simulink model "BLDC_120deg_calibration_routine"  (R2024a)
settings: Solver=ode15s  StartTime=0.0  StopTime=2.25  RelTol=1e-3
model workspace (MAT data in the model file):
  t = 3
values from neighbouring files (symbols this model uses):
  D_m = 1e-3    (= 0.001)    [BLDC_Parameters.m]
  J_t = 1e-3    (= 0.001)    [BLDC_Parameters.m]
  L_ss = tau_s * r_s    (= 0.0003657)    [BLDC_Parameters.m]
  lambda_m = torque_const/(3*P/4)    (= 0.00985)    [BLDC_Parameters.m]
  P = 8    [BLDC_Parameters.m]
  r_s = r_pp/2    (= 0.345)    [BLDC_Parameters.m]
  R_vs = 1e6    (= 1000000)    [BLDC_Parameters.m]
  state1_tau = -1*mean(out.tau_state_1(end-5:end))*omega    [filter.m]
  state2_tau = -1*mean(out.tau_state_2(end-5:end))*omega    [filter.m]
  state3_tau = -1*mean(out.tau_state_3(end-5:end))*omega    [filter.m]
  state4_tau = -1*mean(out.tau_state_4(end-5:end))*omega    [filter.m]
  state5_tau = -1*mean(out.tau_state_5(end-5:end))*omega    [filter.m]
  state6_tau = -1*mean(out.tau_state_6(end-5:end))*omega    [filter.m]
  tau_s = 1.06e-3    (= 0.00106)    [BLDC_Parameters.m]
  V_bus = 12    [BLDC_Parameters.m]
undefined symbols (not defined in the file or in its folder): DiscIntNeverNeededParam, HallError1, HallError2, HallError3, WrappedHallError1
libraries: simulink x17, dspstat3 x6, spsMosfetLib x6, dspswit3 x5, spsSeriesRLCBranchLib x4, spsVoltageMeasurementLib x3, spsControlledCurrentSourceLib x3, slpidlib x1, spsPWMGeneratorDCDCLib x1, spsDCVoltageSourceLib x1, sps_lib x1
(part 1 of 2)
settings Model: Creator=matthewhasman  LastModifiedBy=matthewhasman

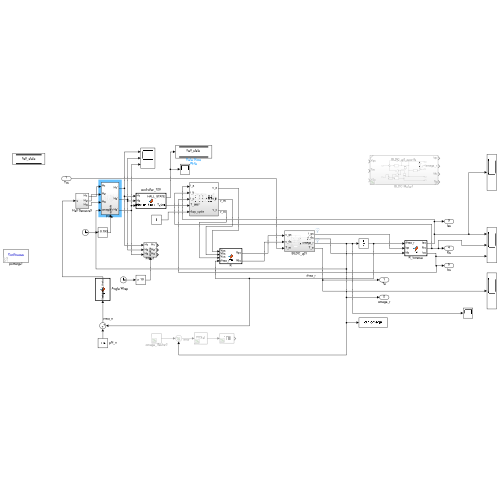
[thumbnail: Simulink's stored preview of the top-level diagram]
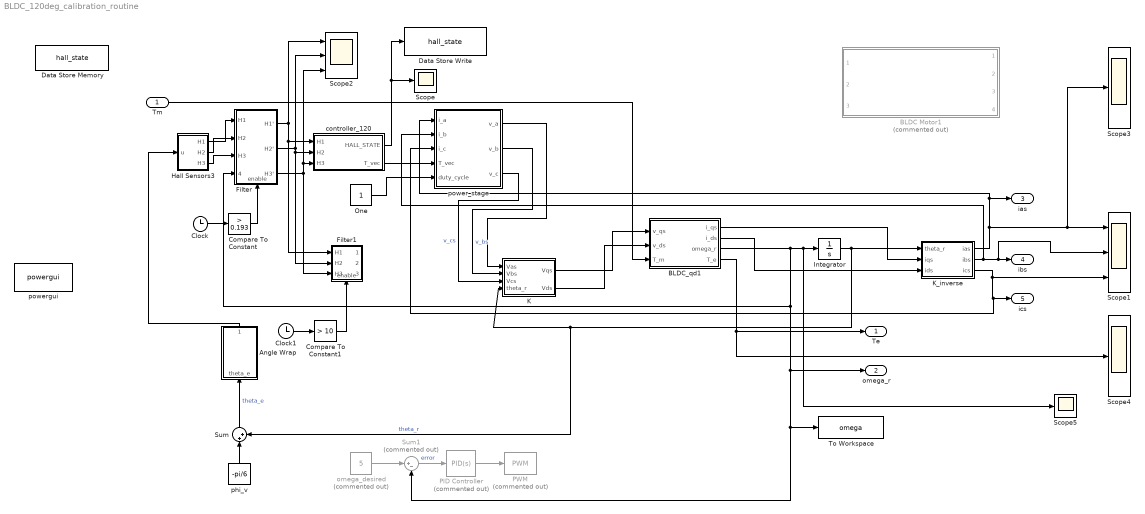
== system BLDC_120deg_calibration_routine ==
  Tm : Inport
  Angle Wrap : MATLAB Function  TreatAsAtomicUnit=on
  BLDC Motor1 : Subsystem  Commented=on  ReferencedSubsystem=BLDC_qd_coords
  BLDC_qd1 : Subsystem
  Clock : Clock
  Clock1 : Clock
  Compare To Constant : simulink/Logic and Bit Operations/Compare To Constant  relop=>  const=0.193  OutDataTypeStr=boolean
  Compare To Constant1 : simulink/Logic and Bit Operations/Compare To Constant  relop=>  const=10  OutDataTypeStr=boolean
  Data Store Memory : DataStoreMemory  DataStoreName=hall_state  WriteAfterWriteMsg=warning  InitialValue=-1  ShowAdditionalParam=off
  Data Store Write : DataStoreWrite  DataStoreName=hall_state  IndexOptions=Index vector (dialog)  Indices=1  OutputSizes=1
  Filter : Subsystem
      settings: PortSchema="{\"entries\":[{\"content\":{\"sides\":[{\"content\":{\"connectorIds\":[\"In1\",\"In2\",\"In3\",\"In4\"]},\"type\":\"ConnectorPlacement.EquallySpacedRectSide\",\"uuid\":\"41cc07ee-628c-4a70-9df5-9f0309ace514\"},{\"content\":{\"connectorIds\":[\"Out1\",\"Out2\",\"Out3\"],\"side\":\"RIGHT\"},\"type\":\"ConnectorPlacement.EquallySpacedRectSide\",\"uuid\":\"f15fe452-14eb-427f-ab3a-fd71ce3a6850\"},{\"content\":{\"side\":\"TOP\"},\"type\":\"ConnectorPlacement.EquallySpacedRectSide\",\"uuid\":\"a8bc91a7-4d9a-483b-b43c-6e71d37ef696\"},{\"content\":{\"connectorIds\":[\"In5\"],\"side\":\"BOTTOM\"},\"type\":\"ConnectorPlacement.EquallySpacedRectSide\",\"uuid\":\"b72df871-072d-40c5-aee7-b72e6fa3c48e\"}]},\"type\":\"ConnectorPlacement.EquallySpacedConnector\",\"uuid\":\"b89763df-ec25-48a8-941f-c6d30f9b0f80\"}],\"packageUris\":[\"http://schema.mathworks.com/mf0/Connector/R2020b\"],\"version\":\"1.0\"}"
  Filter1 : Subsystem
      settings: PortSchema="{\"entries\":[{\"content\":{\"sides\":[{\"content\":{\"connectorIds\":[\"In1\",\"In2\",\"In3\"]},\"type\":\"ConnectorPlacement.EquallySpacedRectSide\",\"uuid\":\"41cc07ee-628c-4a70-9df5-9f0309ace514\"},{\"content\":{\"connectorIds\":[\"Out1\",\"Out2\",\"Out3\"],\"side\":\"RIGHT\"},\"type\":\"ConnectorPlacement.EquallySpacedRectSide\",\"uuid\":\"f15fe452-14eb-427f-ab3a-fd71ce3a6850\"},{\"content\":{\"side\":\"TOP\"},\"type\":\"ConnectorPlacement.EquallySpacedRectSide\",\"uuid\":\"a8bc91a7-4d9a-483b-b43c-6e71d37ef696\"},{\"content\":{\"connectorIds\":[\"In4\"],\"side\":\"BOTTOM\"},\"type\":\"ConnectorPlacement.EquallySpacedRectSide\",\"uuid\":\"b72df871-072d-40c5-aee7-b72e6fa3c48e\"}]},\"type\":\"ConnectorPlacement.EquallySpacedConnector\",\"uuid\":\"b89763df-ec25-48a8-941f-c6d30f9b0f80\"}],\"packageUris\":[\"http://schema.mathworks.com/mf0/Connector/R2020b\"],\"version\":\"1.0\"}"
  Hall Sensors3 : Subsystem
  Integrator : Integrator
  K : MATLAB Function  TreatAsAtomicUnit=on
  K_inverse : MATLAB Function  TreatAsAtomicUnit=on
  One : Constant  OutDataTypeStr=Inherit: Inherit via back propagation
  PID Controller : slpidlib/PID Controller  Commented=on  Controller=PID  Form=Parallel  TimeDomain=Continuous-time  UseExternalTs=off  SampleTime=-1  IntegratorMethod=Forward Euler  FilterMethod=Forward Euler  ControllerParametersSource=internal  P=8  I=5  UseKiTs=off  D=1  UseExternalDerivativeSource=off  N=100  UseFilter=on  TunerSelectOption=Transfer Function Based (PID Tuner App)  InitialConditionSource=internal  InitialConditionForIntegrator=0  InitialConditionForFilter=0  DifferentiatorICPrevScaledInput=0  ExternalReset=none  TrackingMode=off  Kt=1  LimitOutput=off  SatLimitsSource=internal  UpperSaturationLimit=inf  LowerSaturationLimit=-inf  LinearizeAsGain=on  AntiWindupMode=none  Kb=1  LimitIntegrator=off  UpperIntegratorSaturationLimit=inf  LowerIntegratorSaturationLimit=-inf  POutMin=[]  POutMax=[]  IOutMin=[]  IOutMax=[]  DOutMin=[]  DOutMax=[]  NOutMin=[]  NOutMax=[]  SumOutMin=[]  SumOutMax=[]  SaturationOutMin=[]  SaturationOutMax=[]  PParamMin=[]  PParamMax=[]  IParamMin=[]  IParamMax=[]  DParamMin=[]  DParamMax=[]  NParamMin=[]  NParamMax=[]  KbParamMin=[]  KbParamMax=[]  KtParamMin=[]  KtParamMax=[]  KbOutMin=[]  KbOutMax=[]  KtOutMin=[]  KtOutMax=[]  IntegratorOutMin=[]  IntegratorOutMax=[]  FilterOutMin=[]  FilterOutMax=[]  SumI1OutMin=[]  SumI1OutMax=[]  SumI2OutMin=[]  SumI2OutMax=[]  SumI3OutMin=[]  SumI3OutMax=[]  SumI4OutMin=[]  SumI4OutMax=[]  SumDOutMin=[]  SumDOutMax=[]  DifferentiatorOutMin=[]  DifferentiatorOutMax=[]  FilterDiffOutCoefMin=[]  FilterDiffOutCoefMax=[]  ReciprocalOutMin=[]  ReciprocalOutMax=[]  SumDenOutMin=[]  SumDenOutMax=[]  SumNumOutMin=[]  SumNumOutMax=[]  DivideOutMin=[]  DivideOutMax=[]  UdiffTsProdOutMin=[]  UdiffTsProdOutMax=[]  NTsProdOutMin=[]  NTsProdOutMax=[]  UintegralTsProdOutMin=[]  UintegralTsProdOutMax=[]  UngainTsProdOutMin=[]  UngainTsProdOutMax=[]  ClampingZeroOutDataTypeStr=Inherit: Inherit via back propagation  ClampingZeroOutMin=[]  ClampingZeroOutMax=[]  FilterDenConstantOutDataTypeStr=Inherit: Inherit via back propagation  FilterDenConstantOutMin=[]  FilterDenConstantOutMax=[]  PCopyOutDataTypeStr=Inherit: Inherit via back propagation  PCopyOutMin=[]  PCopyOutMax=[]  NCopyOutDataTypeStr=Inherit: Inherit via back propagation  NCopyOutMin=[]  NCopyOutMax=[]  IntegratorContinuousStateAttributes=''  IntegratorStateMustResolveToSignalObject=off  IntegratorRTWStateStorageClass=Auto  FilterContinuousStateAttributes=''  FilterStateMustResolveToSignalObject=off  FilterRTWStateStorageClass=Auto  ParallelPVariant=InternalParameters  IdealPVariant=Disabled  IVariant=InternalParameters  DVariant=InternalParameters  IntegratorVariant=Continuous  SatVariant=Disabled  AWVariant=Passthrough  PCopyVariant=Disabled  TRVariant=Disabled  FdbkBlocksVariant=Forward  IdealPFdbkVariant=Disabled  SatFdbkVariant=Disabled  DerivativeFilterVariant=ContFilter  NVariant=InternalParameters  NCopyVariant=Disabled  FilterICVariant=InternalICsFilter  IntegratorICVariant=InternalICs  ExternalResetVariant=Disabled  TRSumVariant=Passthrough  SumFdbkVariant=Disabled  SumVariant=Sum_PID  TsampFilterVariant=InternalTs  TsampNgainVariant=Passthrough  TsampIntegralVariant=Disabled_SignalSpec  ExternalSaturationOutDataTypeStr=Inherit: Same as second input  DerivativeSourceVariant=ErrorSignal
  PWM : simulink/Discontinuities/PWM  Commented=on  DisableCoverage=on  Period=0.0001  InitialDelay=0  DisallowZeroDutyCycle=off  RunAtFixedTimeIntervals=off  SampleTime=0.1
  Scope{,3..5} (4 alike) : Scope
  Scope1 : Scope  NumInputPorts=3
  Scope2 : Scope  NumInputPorts=3
  Sum : Sum  Inputs=|++
  Sum1 : Sum  Commented=on  Inputs=|+-
  To Workspace : ToWorkspace  VariableName=omega  SampleTime=-1
  controller_120 : MATLAB Function  TreatAsAtomicUnit=on
  omega_desired : Constant  Commented=on  Value=5
  phi_v : Constant  Value=-pi/6
  power_stage : Subsystem
  powergui : sps_lib/powergui  Priority=1  SimulationMode=Continuous  SampleTime=50e-6  frequency=60  Iterations=50  frequencyindice=0  Pbase=100e6  ErrMax=1e-4  UnitsV=kV  UnitsW=MW  buscounter=0  FunctionMessages=off  echomessages=off  EnableUseOfTLC=off  CurrentSourceSwitches=off  DisableSnubberDevices=off  DisableRonSwitches=off  DisableVfSwitches=off  DisplayEquations=off  AutomaticDiscreteSolvers=off  SolverType=Tustin/Backward Euler (TBE)  Interpol=off  ExternalGateDelay=off  methode=off  Ts=100  x0status=blocks  SPID=on  SwTol=0  HookPort=off  NonlinearTolerance=1e-4  nMaxIteration=100  ContinueOnMaxIteration=off  RestoreLinks=warning  ResistiveCurrentMeasurement=off  Frange=[0:2:500]  Ylog=off  Xlog=on  ShowGrid=off  save=off  variable=ZData  structure=0  ZoomFFT=off  StartTime=0.0  cycles=1  DisplayStyle=1  fundamental=60  FreqAxis=off  MaxFrequency=1000  frequencyindicesteady=1  RmsSteady=1  display=off
  Te : Outport
  omega_r : Outport  Port=2
  ias : Outport  Port=3
  ibs : Outport  Port=4
  ics : Outport  Port=5
  wires:
  Integrator/1 -> K_inverse/1(theta_r), K/4(theta_r), Sum/2  "theta_r"
  BLDC_qd1/1(i_qs) -> K_inverse/2(iqs)
  BLDC_qd1/2(i_ds) -> K_inverse/3(ids)
  K/1(Vqs) -> BLDC_qd1/1(v_qs)
  Tm/1 -> BLDC_qd1/3(T_m)
  phi_v/1 -> Sum/1
  omega_desired/1 -> Sum1/1
  Sum1/1 -> PID Controller/1  "error"
  PID Controller/1 -> PWM/1
  K/2(Vds) -> BLDC_qd1/2(v_ds)
  Sum/1 -> Angle Wrap/1(theta_e)  "theta_e"
  BLDC_qd1/3(omega_r) -> Filter/4(omega_r), omega_r/1, To Workspace/1, Sum1/2, Scope5/1, Integrator/1
  BLDC_qd1/4(T_e) -> Scope4/1, Te/1
  K_inverse/1(ias) -> ias/1, power_stage/1(i_a), Scope3/1, Scope1/1
  K_inverse/2(ibs) -> power_stage/2(i_b), Scope1/2, ibs/1
  K_inverse/3(ics) -> power_stage/3(i_c), ics/1, Scope1/3
  controller_120/2(T_vec) -> power_stage/4(T_vec)
  power_stage/1(v_a) -> K/1(Vas)
  power_stage/2(v_b) -> K/2(Vbs)  "v_bs"
  power_stage/3(v_c) -> K/3(Vcs)  "v_cs"
  Angle Wrap/1(wrapped_theta) -> Hall Sensors3/1(u)
  Hall Sensors3/1(H1) -> Filter/1(H1)
  Hall Sensors3/2(H2) -> Filter/2(H2)
  Hall Sensors3/3(H3) -> Filter/3(H3)
  Compare To Constant/1 -> Filter/5(enable)
  Filter/1(H1') -> Scope2/1, Filter1/1(H1), controller_120/1(H1)
  Filter/2(H2') -> Scope2/2, Filter1/2(H2), controller_120/2(H2)
  Filter/3(H3') -> Scope2/3, controller_120/3(H3), Filter1/3(H3)
  Clock/1 -> Compare To Constant/1
  controller_120/1(HALL_STATE) -> Scope/1, Data Store Write/1
  One/1 -> power_stage/5(duty_cycle)
  Compare To Constant1/1 -> Filter1/4(enable)
  Clock1/1 -> Compare To Constant1/1

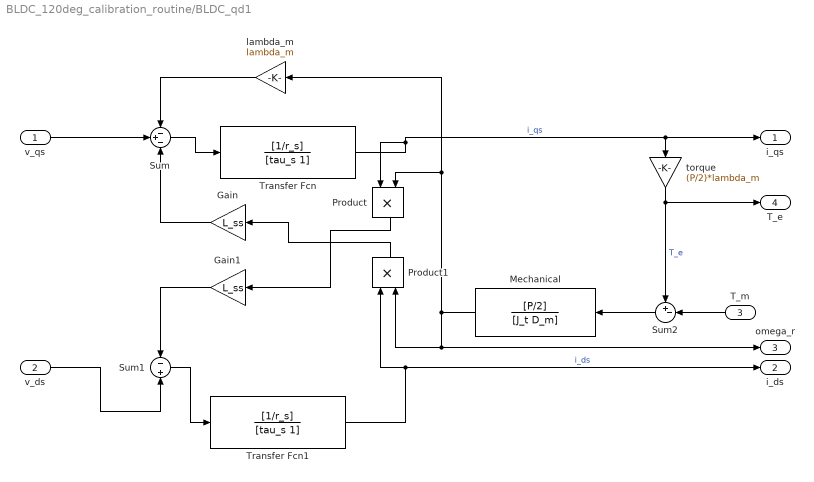
== system BLDC_120deg_calibration_routine/BLDC_qd1 ==
  v_qs : Inport
  v_ds : Inport  Port=2
  T_m : Inport  Port=3
  Gain : Gain  Gain=L_ss
  Gain1 : Gain  Gain=L_ss
  Mechanical : TransferFcn  Numerator=[P/2]  Denominator=[J_t D_m]
  Product : Product
  Product1 : Product
  Sum : Sum  Inputs=-+-
  Sum1 : Sum  Inputs=-+
  Sum2 : Sum  Inputs=+-|
  Transfer Fcn : TransferFcn  Numerator=[1/r_s]  Denominator=[tau_s 1]
  Transfer Fcn1 : TransferFcn  Numerator=[1/r_s]  Denominator=[tau_s 1]
  lambda_m : Gain  Gain=lambda_m
  torque : Gain  Gain=(P/2)*lambda_m
  i_qs : Outport
  i_ds : Outport  Port=2
  omega_r : Outport  Port=3
  T_e : Outport  Port=4
  wires:
  T_m/1 -> Sum2/2
  Sum1/1 -> Transfer Fcn1/1
  Gain1/1 -> Sum1/1
  Product1/1 -> Gain/1
  Transfer Fcn1/1 -> i_ds/1, Product1/1  "i_ds"
  Mechanical/1 -> lambda_m/1, Product/2, omega_r/1, Product1/2
  torque/1 -> T_e/1, Sum2/1  "T_e"
  v_ds/1 -> Sum1/2
  Transfer Fcn/1 -> i_qs/1, torque/1, Product/1  "i_qs"
  Product/1 -> Gain1/1
  Gain/1 -> Sum/3
  v_qs/1 -> Sum/2
  Sum/1 -> Transfer Fcn/1
  Sum2/1 -> Mechanical/1
  lambda_m/1 -> Sum/1

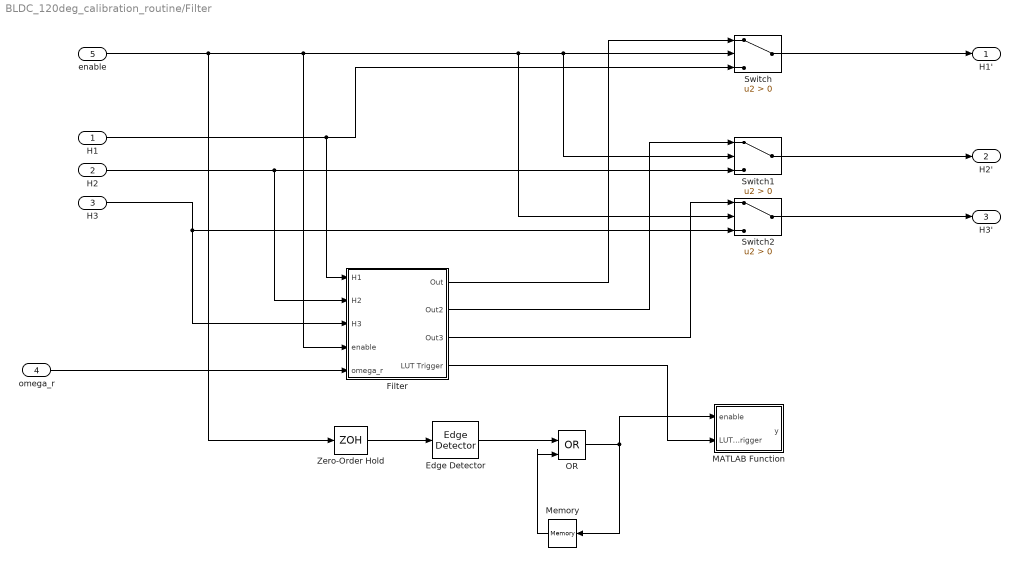
== system BLDC_120deg_calibration_routine/Filter ==
  H1 : Inport
  H2 : Inport  Port=2
  H3 : Inport  Port=3
  omega_r : Inport  Port=4
  enable : Inport  Port=5
  Edge Detector : dspswit3/Edge Detector  InputProcessing=Columns as channels (frame based)
  Filter : Subsystem
  MATLAB Function : MATLAB Function  TreatAsAtomicUnit=on
  Memory : Memory
  OR : Logic  Operator=OR  IconShape=distinctive  AllPortsSameDT=off  OutDataTypeStr=boolean
  Switch : Switch  Criteria=u2 > Threshold  SaturateOnIntegerOverflow=off  InputSameDT=off
  Switch1 : Switch  Criteria=u2 > Threshold  SaturateOnIntegerOverflow=off  InputSameDT=off
  Switch2 : Switch  Criteria=u2 > Threshold  SaturateOnIntegerOverflow=off  InputSameDT=off
  Zero-Order Hold : ZeroOrderHold  SampleTime=-1
  H1' : Outport
  H2' : Outport  Port=2
  H3' : Outport  Port=3
  wires:
  H1/1 -> Switch/3, Filter/1(H1)
  H2/1 -> Filter/2(H2), Switch1/3
  H3/1 -> Switch2/3, Filter/3(H3)
  enable/1 -> Switch2/2, Switch1/2, Switch/2, Filter/4(enable), Zero-Order Hold/1
  Switch/1 -> H1'/1
  Switch1/1 -> H2'/1
  Switch2/1 -> H3'/1
  Filter/1(Out) -> Switch/1
  Filter/2(Out2) -> Switch1/1
  Filter/3(Out3) -> Switch2/1
  omega_r/1 -> Filter/5(omega_r)
  Edge Detector/1 -> OR/1
  Zero-Order Hold/1 -> Edge Detector/1
  OR/1 -> MATLAB Function/1(enable), Memory/1
  Memory/1 -> OR/2
  Filter/4(LUT Trigger) -> MATLAB Function/2(LUT_Trigger)

== system BLDC_120deg_calibration_routine/Filter1 ==
  H1 : Inport
  H2 : Inport  Port=2
  H3 : Inport  Port=3
  enable : Inport  Port=4
  Filter : Subsystem
  Switch : Switch  Criteria=u2 > Threshold  SaturateOnIntegerOverflow=off  InputSameDT=off
  Switch1 : Switch  Criteria=u2 > Threshold  SaturateOnIntegerOverflow=off  InputSameDT=off
  Switch2 : Switch  Criteria=u2 > Threshold  SaturateOnIntegerOverflow=off  InputSameDT=off
  H1' : Outport
  H2' : Outport  Port=2
  H3' : Outport  Port=3
  wires:
  H1/1 -> Switch/3, Filter/1(H1)
  H2/1 -> Filter/2(H2), Switch1/3
  H3/1 -> Switch2/3, Filter/3(H3)
  enable/1 -> Filter/4(enable), Switch2/2, Switch1/2, Switch/2
  Switch/1 -> H1'/1
  Switch1/1 -> H2'/1
  Switch2/1 -> H3'/1
  Filter/1(Out) -> Switch/1
  Filter/2(Out2) -> Switch1/1
  Filter/3(Out3) -> Switch2/1

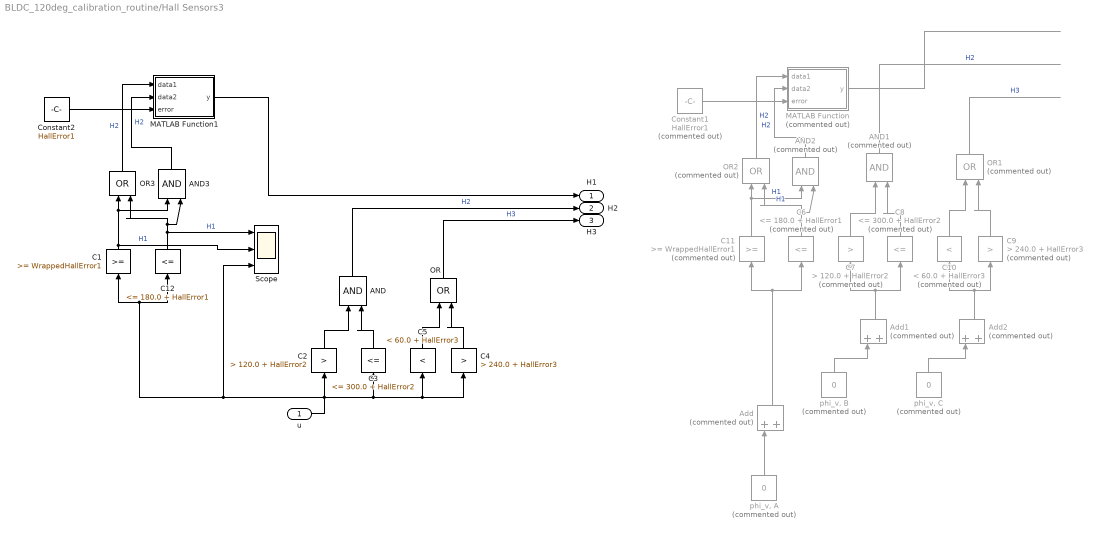
== system BLDC_120deg_calibration_routine/Hall Sensors3 ==
  u : Inport
  AND : Logic  IconShape=distinctive  AllPortsSameDT=off  OutDataTypeStr=boolean
  AND1 : Logic  Commented=on  IconShape=distinctive  AllPortsSameDT=off  OutDataTypeStr=boolean
  AND2 : Logic  Commented=on  IconShape=distinctive  AllPortsSameDT=off  OutDataTypeStr=boolean
  AND3 : Logic  IconShape=distinctive  AllPortsSameDT=off  OutDataTypeStr=boolean
  Add : Sum  Commented=on
  Add1 : Sum  Commented=on
  Add2 : Sum  Commented=on
  C1 : simulink/Logic and Bit Operations/Compare To Constant  relop=>=  const=WrappedHallError1  OutDataTypeStr=boolean
  C10 : simulink/Logic and Bit Operations/Compare To Constant  Commented=on  relop=<  const=60.0 + HallError3  OutDataTypeStr=boolean
  C11 : simulink/Logic and Bit Operations/Compare To Constant  Commented=on  relop=>=  const=WrappedHallError1  OutDataTypeStr=boolean
  C12 : simulink/Logic and Bit Operations/Compare To Constant  relop=<=  const=180.0 + HallError1  OutDataTypeStr=boolean
  C2 : simulink/Logic and Bit Operations/Compare To Constant  relop=>  const=120.0 + HallError2  OutDataTypeStr=boolean
  C3 : simulink/Logic and Bit Operations/Compare To Constant  relop=<=  const=300.0 + HallError2  OutDataTypeStr=boolean
  C4 : simulink/Logic and Bit Operations/Compare To Constant  relop=>  const=240.0 + HallError3  OutDataTypeStr=boolean
  C5 : simulink/Logic and Bit Operations/Compare To Constant  relop=<  const=60.0 + HallError3  OutDataTypeStr=boolean
  C6 : simulink/Logic and Bit Operations/Compare To Constant  Commented=on  relop=<=  const=180.0 + HallError1  OutDataTypeStr=boolean
  C7 : simulink/Logic and Bit Operations/Compare To Constant  Commented=on  relop=>  const=120.0 + HallError2  OutDataTypeStr=boolean
  C8 : simulink/Logic and Bit Operations/Compare To Constant  Commented=on  relop=<=  const=300.0 + HallError2  OutDataTypeStr=boolean
  C9 : simulink/Logic and Bit Operations/Compare To Constant  Commented=on  relop=>  const=240.0 + HallError3  OutDataTypeStr=boolean
  Constant1 : Constant  Commented=on  Value=HallError1
  Constant2 : Constant  Value=HallError1
  MATLAB Function : MATLAB Function  Commented=on  TreatAsAtomicUnit=on
  MATLAB Function1 : MATLAB Function  TreatAsAtomicUnit=on
  OR : Logic  Operator=OR  IconShape=distinctive  AllPortsSameDT=off  OutDataTypeStr=boolean
  OR1 : Logic  Commented=on  Operator=OR  IconShape=distinctive  AllPortsSameDT=off  OutDataTypeStr=boolean
  OR2 : Logic  Commented=on  Operator=OR  IconShape=distinctive  AllPortsSameDT=off  OutDataTypeStr=boolean
  OR3 : Logic  Operator=OR  IconShape=distinctive  AllPortsSameDT=off  OutDataTypeStr=boolean
  Scope : Scope  NumInputPorts=3
  "phi_v, A" : Constant  Commented=on  Value=0
  "phi_v, B" : Constant  Commented=on  Value=0
  "phi_v, C" : Constant  Commented=on  Value=0
  H1 : Outport
  H2 : Outport  Port=2
  H3 : Outport  Port=3
  wires:
  C5/1 -> OR/1
  AND/1 -> H2/1  "H2"
  C4/1 -> OR/2
  C3/1 -> AND/2
  C2/1 -> AND/1
  OR/1 -> H3/1  "H3"
  Add1/1 -> C8/1, C7/1
  "phi_v, C"/1 -> Add2/1
  "phi_v, B"/1 -> Add1/1
  C10/1 -> OR1/1
  ? -> Add2/2, Add1/2, Add/2
  OR2/1 -> MATLAB Function/1(data1)  "H2"
  "phi_v, A"/1 -> Add/1
  C9/1 -> OR1/2
  Add/1 -> C6/1, C11/1
  C7/1 -> AND1/1
  Add2/1 -> C10/1, C9/1
  Constant1/1 -> MATLAB Function/3(error)
  OR1/1 -> ?  "H3"
  AND1/1 -> ?  "H2"
  C6/1 -> AND2/2, OR2/2  "H1"
  AND2/1 -> MATLAB Function/2(data2)  "H2"
  MATLAB Function/1(y) -> ?
  C11/1 -> AND2/1, OR2/1  "H1"
  C8/1 -> AND1/2
  u/1 -> Scope/3, C12/1, C1/1, C2/1, C5/1, C4/1, C3/1
  OR3/1 -> MATLAB Function1/1(data1)  "H2"
  Constant2/1 -> MATLAB Function1/3(error)
  C1/1 -> AND3/1, OR3/1, Scope/2  "H1"
  C12/1 -> AND3/2, OR3/2, Scope/1  "H1"
  AND3/1 -> MATLAB Function1/2(data2)  "H2"
  MATLAB Function1/1(y) -> H1/1

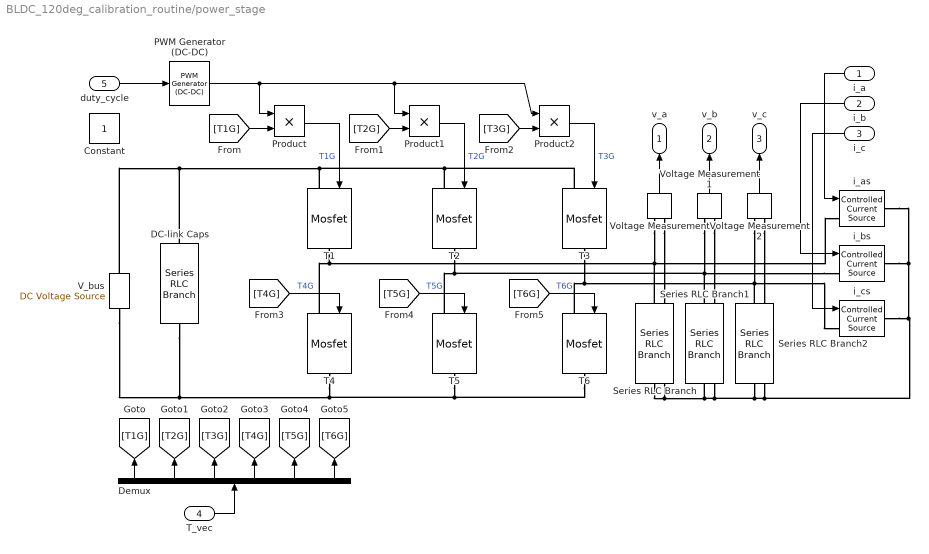
== system BLDC_120deg_calibration_routine/power_stage ==
  i_a : Inport
  i_b : Inport  Port=2
  i_c : Inport  Port=3
  T_vec : Inport  Port=4
  duty_cycle : Inport  Port=5
  Constant : Constant
  DC-link Caps : spsSeriesRLCBranchLib/Series RLC Branch  LConnTagsString=__new0  RConnTagsString=__new0  BranchType=RC  Resistance=1e-6  Inductance=0  SetiL0=off  InitialCurrent=0  Capacitance=100e-6  Setx0=off  InitialVoltage=0  Measurements=None
  Demux : Demux  Outputs=6
  PWM Generator (DC-DC) : spsPWMGeneratorDCDCLib/PWM Generator (DC-DC)  Fsw=f_SW_Hz  Ts=0
  Product : Product
  Product1 : Product
  Product2 : Product
  Series RLC Branch : spsSeriesRLCBranchLib/Series RLC Branch  LConnTagsString=__new0  RConnTagsString=__new0  BranchType=R  Resistance=R_vs  Inductance=0  SetiL0=off  InitialCurrent=0  Capacitance=inf  Setx0=off  InitialVoltage=0  Measurements=None
  Series RLC Branch1 : spsSeriesRLCBranchLib/Series RLC Branch  LConnTagsString=__new0  RConnTagsString=__new0  BranchType=R  Resistance=R_vs  Inductance=0  SetiL0=off  InitialCurrent=0  Capacitance=inf  Setx0=off  InitialVoltage=0  Measurements=None
  Series RLC Branch2 : spsSeriesRLCBranchLib/Series RLC Branch  LConnTagsString=__new0  RConnTagsString=__new0  BranchType=R  Resistance=R_vs  Inductance=0  SetiL0=off  InitialCurrent=0  Capacitance=inf  Setx0=off  InitialVoltage=0  Measurements=None
  T{1..6} (6 alike) : spsMosfetLib/Mosfet  Ron=R_dsON_Ohm  Lon=0  Rd=0.01  Vfd=0.7  IC=0  Rs=1e5  Cs=inf  Measurements=off
  V_bus : spsDCVoltageSourceLib/DC Voltage Source  Amplitude=V_bus  Measurements=None
  Voltage Measurement : spsVoltageMeasurementLib/Voltage Measurement  PhasorSimulation=off  OutputType=Complex  PSBequivalent=0
  Voltage Measurement1 : spsVoltageMeasurementLib/Voltage Measurement  PhasorSimulation=off  OutputType=Complex  PSBequivalent=0
  Voltage Measurement2 : spsVoltageMeasurementLib/Voltage Measurement  PhasorSimulation=off  OutputType=Complex  PSBequivalent=0
  i_as : spsControlledCurrentSourceLib/Controlled Current Source  Initialize=on  Source_Type=AC  Amplitude=0  Phase=0  Frequency=0  Measurements=None
  i_bs : spsControlledCurrentSourceLib/Controlled Current Source  Initialize=on  Source_Type=AC  Amplitude=0  Phase=0  Frequency=0  Measurements=None
  i_cs : spsControlledCurrentSourceLib/Controlled Current Source  Initialize=on  Source_Type=AC  Amplitude=0  Phase=0  Frequency=0  Measurements=None
  v_a : Outport
  v_b : Outport  Port=2
  v_c : Outport  Port=3
  wires:
  T_vec/1 -> Demux/1
  Product1/1 -> T2/1  "T2G"
  PWM Generator (DC-DC)/1 -> Product/1, Product2/1, Product1/1
  Demux/6 -> [T6G]
  [T4G] -> T4/1  "T4G"
  [T5G] -> T5/1  "T5G"
  Demux/4 -> [T4G]
  Voltage Measurement/1 -> v_a/1
  [T2G] -> Product1/2
  Voltage Measurement1/1 -> v_b/1
  Voltage Measurement2/1 -> v_c/1
  i_a/1 -> i_as/1
  Demux/1 -> [T1G]
  Demux/5 -> [T5G]
  [T6G] -> T6/1  "T6G"
  i_c/1 -> i_cs/1
  Product/1 -> T1/1  "T1G"
  [T3G] -> Product2/2
  i_b/1 -> i_bs/1
  Product2/1 -> T3/1  "T3G"
  Demux/2 -> [T2G]
  Demux/3 -> [T3G]
  [T1G] -> Product/2
  duty_cycle/1 -> PWM Generator (DC-DC)/1
  connections:
  i_bs/LConn1 -- Voltage Measurement1/LConn1 -- Series RLC Branch1/LConn1 -- T2/RConn1 -- T5/LConn1
  DC-link Caps/RConn1 -- V_bus/LConn1 -- T4/RConn1 -- T6/RConn1 -- T5/RConn1
  DC-link Caps/LConn1 -- V_bus/RConn1 -- T1/LConn1 -- T3/LConn1 -- T2/LConn1
  T4/LConn1 -- T1/RConn1 -- Voltage Measurement/LConn1 -- Series RLC Branch/LConn1 -- i_as/LConn1
  T3/RConn1 -- T6/LConn1 -- Voltage Measurement2/LConn1 -- Series RLC Branch2/LConn1 -- i_cs/LConn1
  Series RLC Branch/RConn1 -- Voltage Measurement/LConn2 -- i_bs/RConn1 -- i_as/RConn1 -- i_cs/RConn1 -- Voltage Measurement2/LConn2 -- Series RLC Branch2/RConn1 -- Voltage Measurement1/LConn2 -- Series RLC Branch1/RConn1

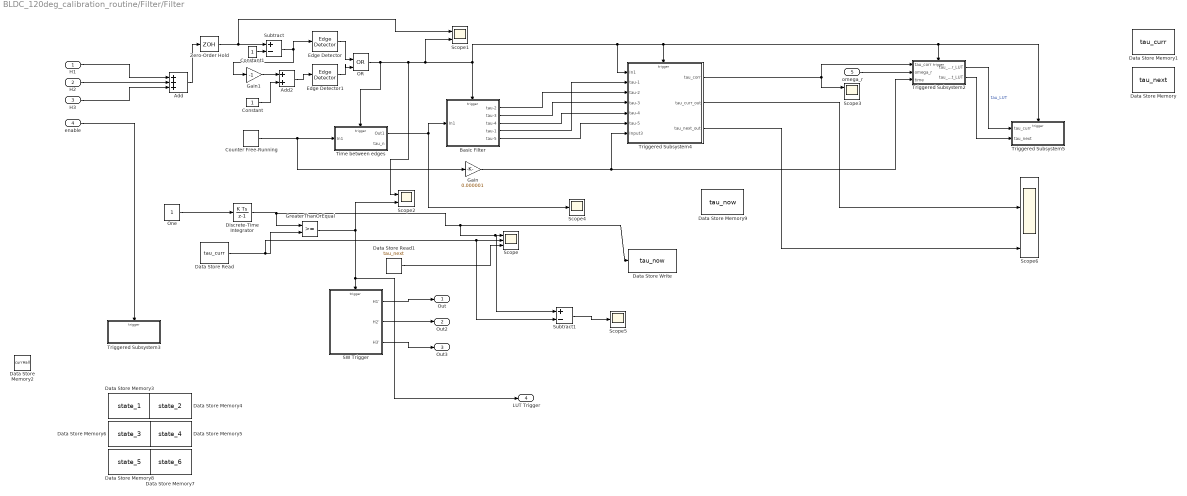
== system BLDC_120deg_calibration_routine/Filter/Filter ==
  H1 : Inport
  H2 : Inport  Port=2
  H3 : Inport  Port=3
  enable : Inport  Port=4
  omega_r : Inport  Port=5
  Add : Sum  Inputs=+++
  Add2 : Sum
  Basic Filter : Subsystem  TreatAsAtomicUnit=on
  Constant : Constant
  Constant1 : Constant
  Counter Free-Running : simulink/Sources/Counter Free-Running  NumBits=32  tsamp=0.000001
  Data Store Memory : DataStoreMemory  DataStoreName=tau_next  WriteAfterWriteMsg=warning  InitialValue=-1  ShowAdditionalParam=off
  Data Store Memory1 : DataStoreMemory  DataStoreName=tau_curr  WriteAfterWriteMsg=warning  InitialValue=0.001  ShowAdditionalParam=off
  Data Store Memory2 : DataStoreMemory  DataStoreName=currHall  WriteAfterWriteMsg=warning  InitialValue=1  ShowAdditionalParam=off
  Data Store Memory3 : DataStoreMemory  DataStoreName=state_1  WriteAfterWriteMsg=warning  ShowAdditionalParam=off
  Data Store Memory4 : DataStoreMemory  DataStoreName=state_2  WriteAfterWriteMsg=warning  ShowAdditionalParam=off
  Data Store Memory5 : DataStoreMemory  DataStoreName=state_4  WriteAfterWriteMsg=warning  ShowAdditionalParam=off
  Data Store Memory6 : DataStoreMemory  DataStoreName=state_3  WriteAfterWriteMsg=warning  ShowAdditionalParam=off
  Data Store Memory7 : DataStoreMemory  DataStoreName=state_6  WriteAfterWriteMsg=warning  ShowAdditionalParam=off
  Data Store Memory8 : DataStoreMemory  DataStoreName=state_5  WriteAfterWriteMsg=warning  ShowAdditionalParam=off
  Data Store Memory9 : DataStoreMemory  DataStoreName=tau_now  WriteAfterWriteMsg=warning  ShowAdditionalParam=off
  Data Store Read : DataStoreRead  DataStoreName=tau_curr  IndexOptions=Index vector (dialog)  Indices=1  OutputSizes=1
  Data Store Read1 : DataStoreRead  DataStoreName=tau_next  IndexOptions=Index vector (dialog)  Indices=1  OutputSizes=1
  Data Store Write : DataStoreWrite  DataStoreName=tau_now  IndexOptions=Index vector (dialog)  Indices=1  OutputSizes=1
  Discrete-Time Integrator : DiscreteIntegrator  SampleTime=1/1e6  ICPrevOutput=DiscIntNeverNeededParam  ICPrevScaledInput=DiscIntNeverNeededParam
  Edge Detector : dspswit3/Edge Detector  InputProcessing=Columns as channels (frame based)
  Edge Detector1 : dspswit3/Edge Detector  InputProcessing=Columns as channels (frame based)
  Gain : Gain  Gain=0.000001
  Gain1 : Gain  Gain=-1
  GreaterThanOrEqual : RelationalOperator  OutDataTypeStr=boolean  RndMeth=Simplest  InputSameDT=off
  OR : Logic  Operator=OR  IconShape=distinctive  AllPortsSameDT=off  OutDataTypeStr=boolean
  One : Constant  OutDataTypeStr=Inherit: Inherit via back propagation
  SW Trigger : Subsystem  Priority=2  TreatAsAtomicUnit=on
  Scope : Scope  NumInputPorts=3
  Scope1 : Scope  NumInputPorts=2
  Scope2 : Scope  NumInputPorts=2
  Scope3 : Scope  NumInputPorts=2
  Scope4 : Scope
  Scope5 : Scope
  Scope6 : Scope  NumInputPorts=4
  Subtract : Sum  Inputs=+-
  Subtract1 : Sum  Inputs=+-
  Time between edges : Subsystem  TreatAsAtomicUnit=on
  Triggered Subsystem2 : Subsystem  TreatAsAtomicUnit=on
  Triggered Subsystem3 : Subsystem  Priority=1  TreatAsAtomicUnit=on
  Triggered Subsystem4 : Subsystem  TreatAsAtomicUnit=on
  Triggered Subsystem5 : Subsystem  TreatAsAtomicUnit=on
  Zero-Order Hold : ZeroOrderHold  SampleTime=0.000001
  Out : Outport
  Out2 : Outport  Port=2
  Out3 : Outport  Port=3
  LUT Trigger : Outport  Port=4
  wires:
  Counter Free-Running/1 -> Gain/1, Time between edges/1(In1)
  Add/1 -> Zero-Order Hold/1
  Time between edges/1(Out1) -> Scope4/1, Basic Filter/1(In1)
  Edge Detector/1 -> OR/1
  Zero-Order Hold/1 -> Scope1/1, Subtract/1
  Subtract/1 -> Edge Detector/1, Gain1/1
  Constant1/1 -> Subtract/2
  Edge Detector1/1 -> OR/2
  Gain1/1 -> Add2/1
  Add2/1 -> Edge Detector1/1
  Constant/1 -> Add2/2
  H1/1 -> Add/1
  H2/1 -> Add/2
  H3/1 -> Add/3
  OR/1 -> Scope2/1, Scope1/2, Triggered Subsystem4/1(In1), Triggered Subsystem2/Trigger, Triggered Subsystem5/Trigger, Triggered Subsystem4/Trigger, Basic Filter/Trigger, Time between edges/Trigger
  Data Store Read/1 -> Subtract1/2, Scope/2, GreaterThanOrEqual/2
  GreaterThanOrEqual/1 -> LUT Trigger/1, SW Trigger/Trigger, Scope2/2
  SW Trigger/3(H3') -> Out3/1
  SW Trigger/2(H2') -> Out2/1
  SW Trigger/1(H1') -> Out/1
  Data Store Read1/1 -> Scope/3
  enable/1 -> Triggered Subsystem3/Trigger
  One/1 -> Discrete-Time Integrator/1
  Discrete-Time Integrator/1 -> Subtract1/1, Scope/1, Data Store Write/1, GreaterThanOrEqual/1
  Triggered Subsystem4/1(tau_corr) -> Triggered Subsystem2/1(tau_corr), Scope3/1
  Basic Filter/1(tau-2) -> Triggered Subsystem4/3(tau-2)
  Basic Filter/2(tau-3) -> Triggered Subsystem4/4(tau-3)
  Basic Filter/3(tau-4) -> Triggered Subsystem4/5(tau-4)
  Gain/1 -> Triggered Subsystem2/3(time), Triggered Subsystem4/7(Input3)
  Basic Filter/4(tau-1) -> Triggered Subsystem4/2(tau-1)
  Basic Filter/5(tau-5) -> Triggered Subsystem4/6(tau-5)
  Subtract1/1 -> Scope5/1
  omega_r/1 -> Triggered Subsystem2/2(omega_r)
  Triggered Subsystem4/2(tau_curr_out) -> Scope6/2
  Triggered Subsystem4/3(tau_next_out) -> Scope6/4
  Triggered Subsystem2/1(tau_curr_LUT) -> Triggered Subsystem5/1(tau_curr)  "tau_LUT"
  Triggered Subsystem2/2(tau_next_LUT) -> Triggered Subsystem5/2(tau_next)

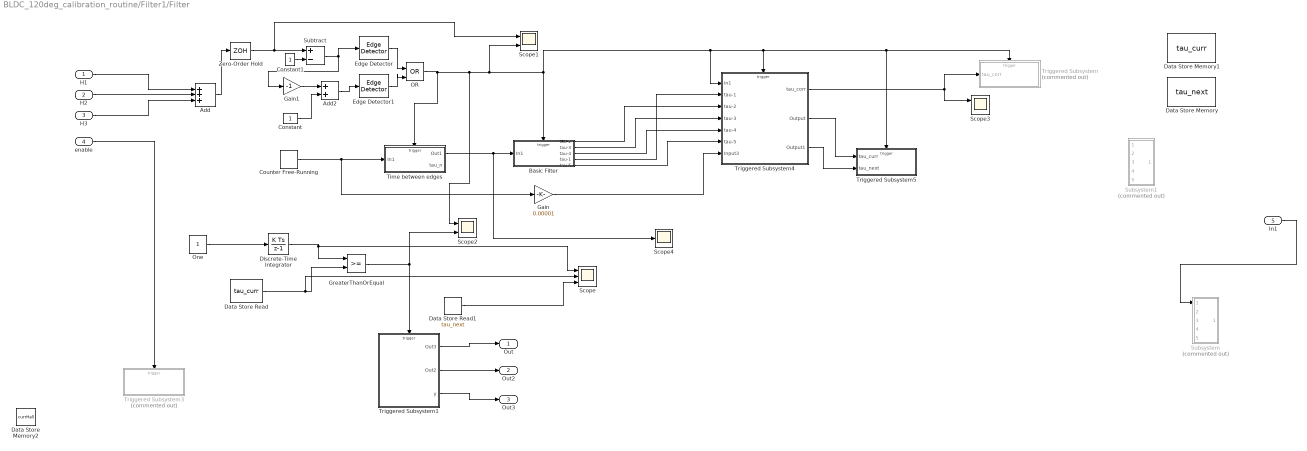
== system BLDC_120deg_calibration_routine/Filter1/Filter ==
  H1 : Inport
  H2 : Inport  Port=2
  H3 : Inport  Port=3
  enable : Inport  Port=4
  In1 : Inport  Port=5
  Add : Sum  Inputs=+++
  Add2 : Sum
  Basic Filter : Subsystem  TreatAsAtomicUnit=on
  Constant : Constant
  Constant1 : Constant
  Counter Free-Running : simulink/Sources/Counter Free-Running  NumBits=32  tsamp=0.000001
  Data Store Memory : DataStoreMemory  DataStoreName=tau_next  WriteAfterWriteMsg=warning  InitialValue=-1  ShowAdditionalParam=off
  Data Store Memory1 : DataStoreMemory  DataStoreName=tau_curr  WriteAfterWriteMsg=warning  InitialValue=0.001  ShowAdditionalParam=off
  Data Store Memory2 : DataStoreMemory  DataStoreName=currHall  WriteAfterWriteMsg=warning  InitialValue=1  ShowAdditionalParam=off
  Data Store Read : DataStoreRead  DataStoreName=tau_curr  IndexOptions=Index vector (dialog)  Indices=1  OutputSizes=1
  Data Store Read1 : DataStoreRead  DataStoreName=tau_next  IndexOptions=Index vector (dialog)  Indices=1  OutputSizes=1
  Discrete-Time Integrator : DiscreteIntegrator  SampleTime=1/1e5  ICPrevOutput=DiscIntNeverNeededParam  ICPrevScaledInput=DiscIntNeverNeededParam
  Edge Detector : dspswit3/Edge Detector  InputProcessing=Columns as channels (frame based)
  Edge Detector1 : dspswit3/Edge Detector  InputProcessing=Columns as channels (frame based)
  Gain : Gain  Gain=0.00001
  Gain1 : Gain  Gain=-1
  GreaterThanOrEqual : RelationalOperator  OutDataTypeStr=boolean  RndMeth=Simplest  InputSameDT=off
  OR : Logic  Operator=OR  IconShape=distinctive  AllPortsSameDT=off  OutDataTypeStr=boolean
  One : Constant  OutDataTypeStr=Inherit: Inherit via back propagation
  Scope : Scope  NumInputPorts=3
  Scope1 : Scope  NumInputPorts=2
  Scope2 : Scope  NumInputPorts=2
  Scope3 : Scope  NumInputPorts=2
  Scope4 : Scope
  Subsystem : Subsystem  Commented=on
  Subsystem1 : Subsystem  Commented=on
  Subtract : Sum  Inputs=+-
  Time between edges : Subsystem  TreatAsAtomicUnit=on
  Triggered Subsystem : Subsystem  Commented=on  TreatAsAtomicUnit=on
  Triggered Subsystem1 : Subsystem  TreatAsAtomicUnit=on
  Triggered Subsystem3 : Subsystem  Commented=on  TreatAsAtomicUnit=on
  Triggered Subsystem4 : Subsystem  TreatAsAtomicUnit=on
  Triggered Subsystem5 : Subsystem  TreatAsAtomicUnit=on
  Zero-Order Hold : ZeroOrderHold  SampleTime=0.0001
  Out : Outport
  Out2 : Outport  Port=2
  Out3 : Outport  Port=3
  wires:
  Counter Free-Running/1 -> Gain/1, Time between edges/1(In1)
  Add/1 -> Zero-Order Hold/1
  Time between edges/1(Out1) -> Scope4/1, Basic Filter/1(In1)
  Edge Detector/1 -> OR/1
  Zero-Order Hold/1 -> Scope1/1, Subtract/1
  Subtract/1 -> Edge Detector/1, Gain1/1
  Constant1/1 -> Subtract/2
  Edge Detector1/1 -> OR/2
  Gain1/1 -> Add2/1
  Add2/1 -> Edge Detector1/1
  Constant/1 -> Add2/2
  H1/1 -> Add/1
  H2/1 -> Add/2
  H3/1 -> Add/3
  OR/1 -> Scope2/1, Scope1/2, Triggered Subsystem4/1(In1), Triggered Subsystem5/Trigger, Triggered Subsystem/Trigger, Triggered Subsystem4/Trigger, Basic Filter/Trigger, Time between edges/Trigger
  Data Store Read/1 -> Scope/2, GreaterThanOrEqual/2
  GreaterThanOrEqual/1 -> Triggered Subsystem1/Trigger, Scope2/2
  Triggered Subsystem1/3(y) -> Out3/1
  Triggered Subsystem1/2(Out2) -> Out2/1
  Triggered Subsystem1/1(Out3) -> Out/1
  Data Store Read1/1 -> Scope/3
  enable/1 -> Triggered Subsystem3/Trigger
  One/1 -> Discrete-Time Integrator/1
  Discrete-Time Integrator/1 -> Scope/1, GreaterThanOrEqual/1
  Triggered Subsystem4/1(tau_corr) -> Scope3/1, Triggered Subsystem/1(tau_corr)
  Basic Filter/1(tau-2) -> Triggered Subsystem4/3(tau-2)
  Basic Filter/2(tau-3) -> Triggered Subsystem4/4(tau-3)
  Basic Filter/3(tau-4) -> Triggered Subsystem4/5(tau-4)
  Gain/1 -> Triggered Subsystem4/7(Input3)
  Triggered Subsystem4/2(Output) -> Triggered Subsystem5/1(tau_curr)
  Triggered Subsystem4/3(Output1) -> Triggered Subsystem5/2(tau_next)
  In1/1 -> Subsystem/1(In1)
  Basic Filter/4(tau-1) -> Triggered Subsystem4/2(tau-1)
  Basic Filter/5(tau-5) -> Triggered Subsystem4/6(tau-5)

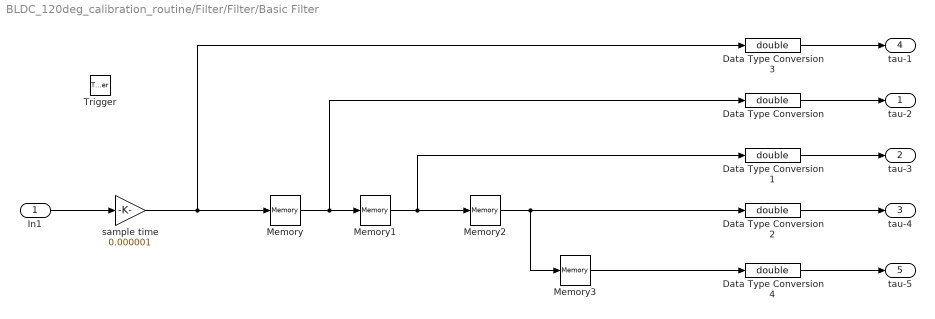
== system BLDC_120deg_calibration_routine/Filter/Filter/Basic Filter ==
  In1 : Inport
  Trigger : TriggerPort  VariantControl=(inherit)
  Data Type Conversion{,1..4} (5 alike) : DataTypeConversion  OutDataTypeStr=double  SaturateOnIntegerOverflow=off  RndMeth=Floor
  Memory{,1..3} (4 alike) : Memory  InheritSampleTime=on
  sample time : Gain  Gain=0.000001
  tau-2 : Outport
  tau-3 : Outport  Port=2
  tau-4 : Outport  Port=3
  tau-1 : Outport  Port=4
  tau-5 : Outport  Port=5
  wires:
  Memory/1 -> Data Type Conversion/1, Memory1/1
  Memory1/1 -> Memory2/1, Data Type Conversion1/1
  In1/1 -> sample time/1
  Data Type Conversion/1 -> tau-2/1
  Data Type Conversion1/1 -> tau-3/1
  Memory2/1 -> Memory3/1, Data Type Conversion2/1
  Data Type Conversion2/1 -> tau-4/1
  sample time/1 -> Data Type Conversion3/1, Memory/1
  Data Type Conversion3/1 -> tau-1/1
  Data Type Conversion4/1 -> tau-5/1
  Memory3/1 -> Data Type Conversion4/1

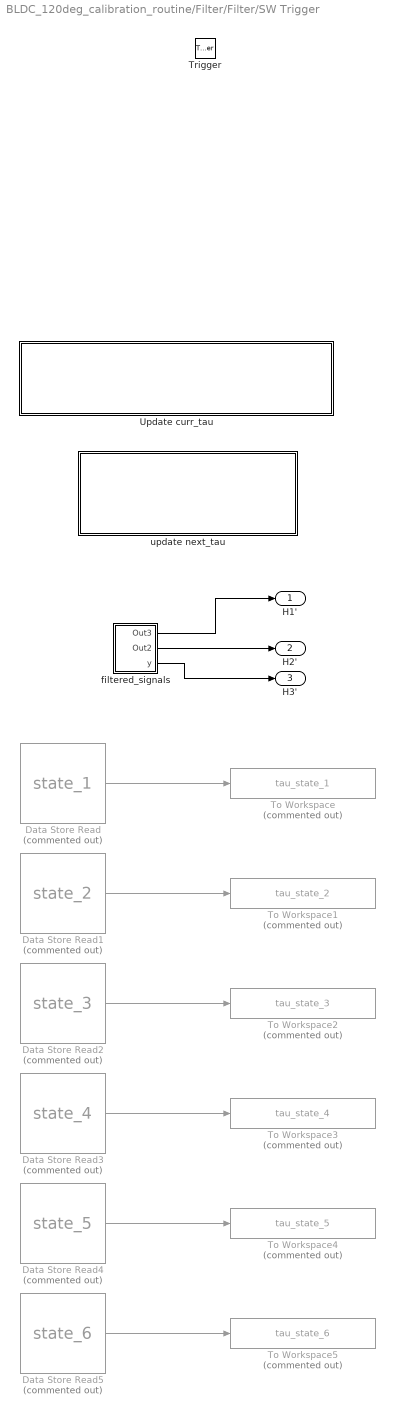
== system BLDC_120deg_calibration_routine/Filter/Filter/SW Trigger ==
  Trigger : TriggerPort  VariantControl=(inherit)
  Data Store Read : DataStoreRead  Commented=on  DataStoreName=state_1  IndexOptions=Index vector (dialog)  Indices=1  OutputSizes=1
  Data Store Read1 : DataStoreRead  Commented=on  DataStoreName=state_2  IndexOptions=Index vector (dialog)  Indices=1  OutputSizes=1
  Data Store Read2 : DataStoreRead  Commented=on  DataStoreName=state_3  IndexOptions=Index vector (dialog)  Indices=1  OutputSizes=1
  Data Store Read3 : DataStoreRead  Commented=on  DataStoreName=state_4  IndexOptions=Index vector (dialog)  Indices=1  OutputSizes=1
  Data Store Read4 : DataStoreRead  Commented=on  DataStoreName=state_5  IndexOptions=Index vector (dialog)  Indices=1  OutputSizes=1
  Data Store Read5 : DataStoreRead  Commented=on  DataStoreName=state_6  IndexOptions=Index vector (dialog)  Indices=1  OutputSizes=1
  To Workspace : ToWorkspace  Commented=on  VariableName=tau_state_1  SampleTime=-1
  To Workspace1 : ToWorkspace  Commented=on  VariableName=tau_state_2  SampleTime=-1
  To Workspace2 : ToWorkspace  Commented=on  VariableName=tau_state_3  SampleTime=-1
  To Workspace3 : ToWorkspace  Commented=on  VariableName=tau_state_4  SampleTime=-1
  To Workspace4 : ToWorkspace  Commented=on  VariableName=tau_state_5  SampleTime=-1
  To Workspace5 : ToWorkspace  Commented=on  VariableName=tau_state_6  SampleTime=-1
  Update curr_tau : Subsystem  Priority=2
  filtered_signals : Subsystem  Priority=4
  update next_tau : Subsystem  Priority=3
  H1' : Outport
  H2' : Outport  Port=2
  H3' : Outport  Port=3
  wires:
  filtered_signals/1(Out3) -> H1'/1
  filtered_signals/2(Out2) -> H2'/1
  filtered_signals/3(y) -> H3'/1
  Data Store Read/1 -> To Workspace/1
  Data Store Read1/1 -> To Workspace1/1
  Data Store Read2/1 -> To Workspace2/1
  Data Store Read3/1 -> To Workspace3/1
  Data Store Read4/1 -> To Workspace4/1
  Data Store Read5/1 -> To Workspace5/1

== system BLDC_120deg_calibration_routine/Filter/Filter/Time between edges ==
  In1 : Inport
  Trigger : TriggerPort  VariantControl=(inherit)
  Gain : Gain  Gain=0.000001
  Memory : Memory  InheritSampleTime=on
  Subtract : Sum  Inputs=+-
  Out1 : Outport
  tau_n : Outport  Port=2
  wires:
  In1/1 -> Gain/1, Subtract/1, Memory/1
  Memory/1 -> Subtract/2
  Subtract/1 -> Out1/1
  Gain/1 -> tau_n/1

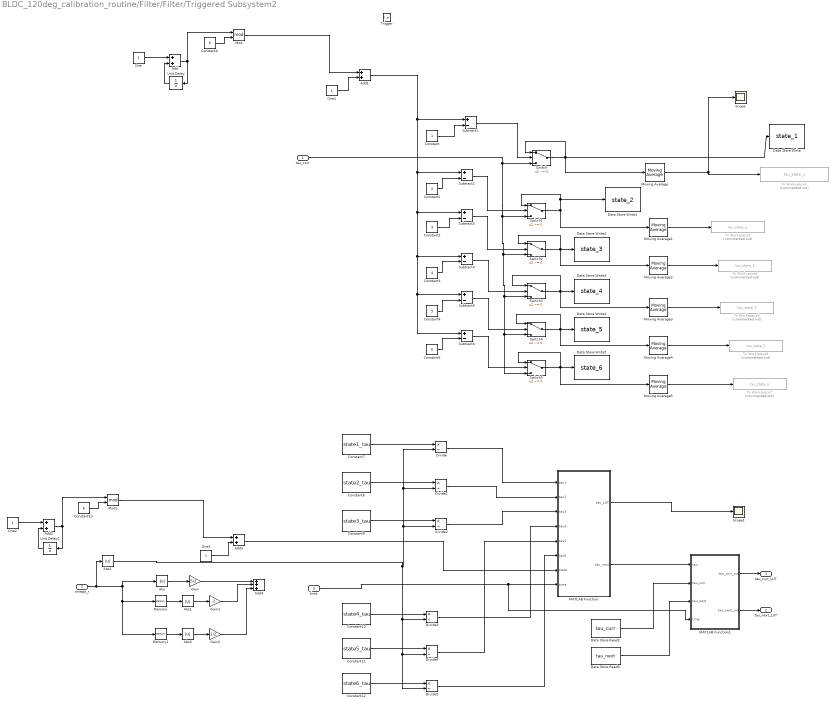
== system BLDC_120deg_calibration_routine/Filter/Filter/Triggered Subsystem2 ==
  tau_corr : Inport
  omega_r : Inport  Port=2
  time : Inport  Port=3
  Trigger : TriggerPort  VariantControl=(inherit)
  Abs{,1..3} (4 alike) : Abs  SaturateOnIntegerOverflow=off
  Add{,1..3} (4 alike) : Sum
  Add4 : Sum  Inputs=+++
  Constant : Constant
  Constant1 : Constant  Value=2
  Constant10 : Constant  Value=state4_tau
  Constant11 : Constant  Value=state5_tau
  Constant12 : Constant  Value=state6_tau
  Constant13 : Constant  Value=6
  Constant2 : Constant  Value=3
  Constant3 : Constant  Value=4
  Constant4 : Constant  Value=5
  Constant5 : Constant  Value=6
  Constant6 : Constant  Value=6
  Constant7 : Constant  Value=state1_tau
  Constant8 : Constant  Value=state2_tau
  Constant9 : Constant  Value=state3_tau
  Data Store Read2 : DataStoreRead  DataStoreName=tau_curr  IndexOptions=Index vector (dialog)  Indices=1  OutputSizes=1
  Data Store Read3 : DataStoreRead  DataStoreName=tau_next  IndexOptions=Index vector (dialog)  Indices=1  OutputSizes=1
  Data Store Write : DataStoreWrite  DataStoreName=state_1  IndexOptions=Index vector (dialog)  Indices=1  OutputSizes=1
  Data Store Write1 : DataStoreWrite  DataStoreName=state_2  IndexOptions=Index vector (dialog)  Indices=1  OutputSizes=1
  Data Store Write2 : DataStoreWrite  DataStoreName=state_3  IndexOptions=Index vector (dialog)  Indices=1  OutputSizes=1
  Data Store Write3 : DataStoreWrite  DataStoreName=state_4  IndexOptions=Index vector (dialog)  Indices=1  OutputSizes=1
  Data Store Write4 : DataStoreWrite  DataStoreName=state_5  IndexOptions=Index vector (dialog)  Indices=1  OutputSizes=1
  Data Store Write5 : DataStoreWrite  DataStoreName=state_6  IndexOptions=Index vector (dialog)  Indices=1  OutputSizes=1
  Divide{,1..5} (6 alike) : Product  Inputs=*/
  Gain : Gain  Gain=5/2
  Gain1 : Gain  Gain=-2
  Gain2 : Gain  Gain=1/2
  MATLAB Function : MATLAB Function  TreatAsAtomicUnit=on
  MATLAB Function1 : MATLAB Function  TreatAsAtomicUnit=on
  Memory : Memory  InheritSampleTime=on
  Memory1 : Memory  InheritSampleTime=on
  Mod : Math  Operator=mod
  Mod1 : Math  Operator=mod
  Moving Average{,1..5} (6 alike) : dspstat3/Moving Average  Method=Exponential weighting  ForgettingFactorPort=off  SpecifyWindowLength=on  WindowLength=100  OverlapLength=3  AllowArbitraryInputLength=off  ForgettingFactor=0.9  SimulateUsing=Interpreted execution
  One{,1..3} (4 alike) : Constant  OutDataTypeStr=Inherit: Inherit via back propagation
  Scope : Scope
  Scope1 : Scope
  Subtract{1..6} (6 alike) : Sum  Inputs=+-
  Switch{,1..5} (6 alike) : Switch  Criteria=u2 ~= 0  SaturateOnIntegerOverflow=off  InputSameDT=off
  To Workspace1 : ToWorkspace  Commented=on  VariableName=tau_state_1  SampleTime=-1
  To Workspace3 : ToWorkspace  Commented=on  VariableName=tau_state_2  SampleTime=-1
  To Workspace4 : ToWorkspace  Commented=on  VariableName=tau_state_3  SampleTime=-1
  To Workspace5 : ToWorkspace  Commented=on  VariableName=tau_state_4  SampleTime=-1
  To Workspace6 : ToWorkspace  Commented=on  VariableName=tau_state_5  SampleTime=-1
  To Workspace7 : ToWorkspace  Commented=on  VariableName=tau_state_6  SampleTime=-1
  Unit Delay : UnitDelay  SampleTime=-1  HasFrameUpgradeWarning=on
  Unit Delay1 : UnitDelay  SampleTime=-1  HasFrameUpgradeWarning=on
  tau_curr_LUT : Outport
  tau_next_LUT : Outport  Port=2
  wires:
  Subtract1/1 -> Switch/2
  Switch1/1 -> Switch1/1, Data Store Write1/1, Moving Average1/1
  Constant/1 -> Subtract1/2
  tau_corr/1 -> Switch/3, Switch1/3, Switch2/3, Switch3/3, Switch5/3, Switch4/3
  Subtract5/1 -> Switch4/2
  Subtract6/1 -> Switch5/2
  Constant5/1 -> Subtract6/2
  Switch4/1 -> Moving Average4/1, Switch4/1, Data Store Write4/1
  Switch/1 -> Switch/1, Data Store Write/1, Moving Average/1
  Switch2/1 -> Moving Average2/1, Switch2/1, Data Store Write2/1
  Constant2/1 -> Subtract3/2
  Constant4/1 -> Subtract5/2
  Constant3/1 -> Subtract4/2
  Constant1/1 -> Subtract2/2
  Switch5/1 -> Moving Average5/1, Switch5/1, Data Store Write5/1
  Subtract4/1 -> Switch3/2
  Subtract3/1 -> Switch2/2
  Switch3/1 -> Moving Average3/1, Switch3/1, Data Store Write3/1
  One/1 -> Add/1
  Add/1 -> Unit Delay/1, Mod/1
  Unit Delay/1 -> Add/2
  Constant6/1 -> Mod/2
  Mod/1 -> Add1/1
  One1/1 -> Add1/2
  Subtract2/1 -> Switch1/2
  Constant7/1 -> Divide/1
  Constant8/1 -> Divide1/1
  Constant9/1 -> Divide2/1
  Constant10/1 -> Divide3/1
  Constant11/1 -> Divide4/1
  Constant12/1 -> Divide5/1
  Divide/1 -> MATLAB Function/1(tau1)
  Divide1/1 -> MATLAB Function/2(tau2)
  Divide2/1 -> MATLAB Function/3(tau3)
  Divide3/1 -> MATLAB Function/4(tau4)
  Divide4/1 -> MATLAB Function/5(tau5)
  Divide5/1 -> MATLAB Function/6(tau6)
  time/1 -> MATLAB Function1/4(time), MATLAB Function/8(time)
  MATLAB Function/2(tau_next) -> MATLAB Function1/1(tau)
  Data Store Read2/1 -> MATLAB Function1/2(tau_curr)
  Data Store Read3/1 -> MATLAB Function1/3(tau_next)
  MATLAB Function1/1(tau_curr_out) -> tau_curr_LUT/1
  MATLAB Function1/2(tau_next_out) -> tau_next_LUT/1
  Add1/1 -> Subtract6/1, Subtract5/1, Subtract4/1, Subtract3/1, Subtract2/1, Subtract1/1
  Moving Average/1 -> Scope/1, To Workspace1/1
  Moving Average1/1 -> To Workspace3/1
  Moving Average2/1 -> To Workspace4/1
  Moving Average3/1 -> To Workspace5/1
  Moving Average4/1 -> To Workspace6/1
  Moving Average5/1 -> To Workspace7/1
  One2/1 -> Add2/1
  Constant13/1 -> Mod1/2
  Add2/1 -> Unit Delay1/1, Mod1/1
  Unit Delay1/1 -> Add2/2
  Mod1/1 -> Add3/1
  One3/1 -> Add3/2
  Add3/1 -> MATLAB Function/7(state)
  MATLAB Function/1(tau_LUT) -> Scope1/1
  Memory/1 -> Abs1/1
  omega_r/1 -> Abs2/1, Abs/1, Memory1/1, Memory/1
  Abs/1 -> Gain/1
  Abs1/1 -> Gain1/1
  Gain1/1 -> Add4/2
  Gain/1 -> Add4/1
  Memory1/1 -> Abs3/1
  Abs3/1 -> Gain2/1
  Gain2/1 -> Add4/3
  Abs2/1 -> Divide5/2, Divide4/2, Divide3/2, Divide/2, Divide1/2, Divide2/2

== system BLDC_120deg_calibration_routine/Filter/Filter/Triggered Subsystem3 ==
  Trigger : TriggerPort  VariantControl=(inherit)
  Constant1 : Constant  Value=6
  Data Store Read : DataStoreRead  DataStoreName=hall_state  IndexOptions=Index vector (dialog)  Indices=1  OutputSizes=1
  Data Store Write : DataStoreWrite  DataStoreName=currHall  IndexOptions=Index vector (dialog)  Indices=1  OutputSizes=1
  MATLAB Function : MATLAB Function  TreatAsAtomicUnit=on
  Scope : Scope
  Scope1 : Scope
  wires:
  Data Store Read/1 -> Scope/1, MATLAB Function/1(u)
  MATLAB Function/1(y) -> Data Store Write/1, Scope1/1

== system BLDC_120deg_calibration_routine/Filter/Filter/Triggered Subsystem4 ==
  In1 : Inport
  tau-1 : Inport  Port=2
  tau-2 : Inport  Port=3
  tau-3 : Inport  Port=4
  tau-4 : Inport  Port=5
  tau-5 : Inport  Port=6
  Input3 : Inport  Port=7
  Trigger : TriggerPort  VariantControl=(inherit)
  Subsystem : Subsystem
  tau_corr : Outport
  tau_curr_out : Outport  Port=2
  tau_next_out : Outport  Port=3
  wires:
  In1/1 -> Subsystem/1(In1)
  Subsystem/1(tau_corr) -> tau_corr/1
  tau-2/1 -> Subsystem/3(tau2)
  tau-3/1 -> Subsystem/4(tau3)
  tau-4/1 -> Subsystem/5(tau4)
  Input3/1 -> Subsystem/7(time)
  Subsystem/2(Output) -> tau_curr_out/1
  Subsystem/3(Output1) -> tau_next_out/1
  tau-1/1 -> Subsystem/2(tau-1)
  tau-5/1 -> Subsystem/6(tau-5)

== system BLDC_120deg_calibration_routine/Filter/Filter/Triggered Subsystem5 ==
  tau_curr : Inport
  tau_next : Inport  Port=2
  Trigger : TriggerPort  VariantControl=(inherit)
  Cast To Double : DataTypeConversion  OutDataTypeStr=double  SaturateOnIntegerOverflow=off  RndMeth=Floor
  Cast To Double1 : DataTypeConversion  OutDataTypeStr=double  SaturateOnIntegerOverflow=off  RndMeth=Floor
  Data Store Write : DataStoreWrite  DataStoreName=tau_curr  IndexOptions=Index vector (dialog)  Indices=1  OutputSizes=1
  Data Store Write1 : DataStoreWrite  DataStoreName=tau_next  IndexOptions=Index vector (dialog)  Indices=1  OutputSizes=1
  wires:
  tau_curr/1 -> Cast To Double/1
  Cast To Double/1 -> Data Store Write/1
  tau_next/1 -> Cast To Double1/1
  Cast To Double1/1 -> Data Store Write1/1

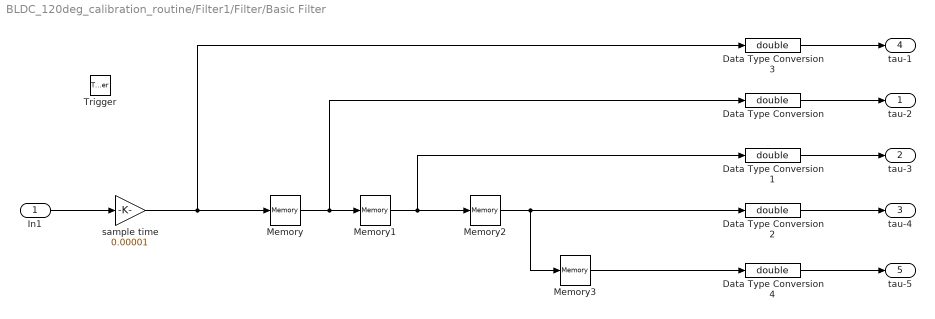
== system BLDC_120deg_calibration_routine/Filter1/Filter/Basic Filter ==
  In1 : Inport
  Trigger : TriggerPort  VariantControl=(inherit)
  Data Type Conversion{,1..4} (5 alike) : DataTypeConversion  OutDataTypeStr=double  SaturateOnIntegerOverflow=off  RndMeth=Floor
  Memory{,1..3} (4 alike) : Memory  InheritSampleTime=on
  sample time : Gain  Gain=0.00001
  tau-2 : Outport
  tau-3 : Outport  Port=2
  tau-4 : Outport  Port=3
  tau-1 : Outport  Port=4
  tau-5 : Outport  Port=5
  wires:
  Memory/1 -> Data Type Conversion/1, Memory1/1
  Memory1/1 -> Memory2/1, Data Type Conversion1/1
  In1/1 -> sample time/1
  Data Type Conversion/1 -> tau-2/1
  Data Type Conversion1/1 -> tau-3/1
  Memory2/1 -> Memory3/1, Data Type Conversion2/1
  Data Type Conversion2/1 -> tau-4/1
  sample time/1 -> Data Type Conversion3/1, Memory/1
  Data Type Conversion3/1 -> tau-1/1
  Data Type Conversion4/1 -> tau-5/1
  Memory3/1 -> Data Type Conversion4/1

== system BLDC_120deg_calibration_routine/Filter1/Filter/Subsystem ==
  In1 : Inport
  tau1 : Inport  Port=2
  tau2 : Inport  Port=3
  tau3 : Inport  Port=4
  time : Inport  Port=5
  Correction Interval : MATLAB Function  Commented=on  TreatAsAtomicUnit=on
  Data Store Read2 : DataStoreRead  Commented=on  DataStoreName=tau_curr  IndexOptions=Index vector (dialog)  Indices=1  OutputSizes=1
  Data Store Read3 : DataStoreRead  Commented=on  DataStoreName=tau_next  IndexOptions=Index vector (dialog)  Indices=1  OutputSizes=1
  MATLAB Function : MATLAB Function  Commented=on  TreatAsAtomicUnit=on
  Scope3 : Scope  Commented=on
  Triggered Subsystem2 : Subsystem  Commented=on  TreatAsAtomicUnit=on
  tau_corr : Outport
  wires:
  tau2/1 -> Correction Interval/2(tau2)
  Data Store Read3/1 -> MATLAB Function/3(tau_next)
  Correction Interval/2(tau_next) -> MATLAB Function/1(tau)
  tau1/1 -> Correction Interval/1(tau1)
  Data Store Read2/1 -> MATLAB Function/2(tau_curr)
  Correction Interval/1(tau_corr) -> tau_corr/1, Scope3/1  "tau_corr"
  MATLAB Function/1(tau_curr_out) -> Triggered Subsystem2/1(tau_curr)
  tau3/1 -> Correction Interval/3(tau3)
  MATLAB Function/2(tau_next_out) -> Triggered Subsystem2/2(tau_next)
  In1/1 -> Triggered Subsystem2/Trigger
  time/1 -> Correction Interval/4(time), MATLAB Function/4(time)

== system BLDC_120deg_calibration_routine/Filter1/Filter/Subsystem1 ==
  In1 : Inport
  tau1 : Inport  Port=2
  tau2 : Inport  Port=3
  tau3 : Inport  Port=4
  time : Inport  Port=5
  Correction Interval : MATLAB Function  TreatAsAtomicUnit=on
  Data Store Read2 : DataStoreRead  DataStoreName=tau_curr  IndexOptions=Index vector (dialog)  Indices=1  OutputSizes=1
  Data Store Read3 : DataStoreRead  DataStoreName=tau_next  IndexOptions=Index vector (dialog)  Indices=1  OutputSizes=1
  MATLAB Function : MATLAB Function  TreatAsAtomicUnit=on
  Scope3 : Scope
  Triggered Subsystem2 : Subsystem  TreatAsAtomicUnit=on
  tau_corr : Outport
  wires:
  tau2/1 -> Correction Interval/2(tau2)
  tau3/1 -> Correction Interval/3(tau3)
  In1/1 -> Triggered Subsystem2/Trigger
  time/1 -> Correction Interval/4(time), MATLAB Function/4(time)
  Data Store Read2/1 -> MATLAB Function/2(tau_curr)
  Data Store Read3/1 -> MATLAB Function/3(tau_next)
  Correction Interval/1(tau_corr) -> tau_corr/1, Scope3/1  "tau_corr"
  MATLAB Function/1(tau_curr_out) -> Triggered Subsystem2/1(tau_curr)
  MATLAB Function/2(tau_next_out) -> Triggered Subsystem2/2(tau_next)
  tau1/1 -> Correction Interval/1(tau1)
  Correction Interval/2(tau_next) -> MATLAB Function/1(tau)

== system BLDC_120deg_calibration_routine/Filter1/Filter/Time between edges ==
  In1 : Inport
  Trigger : TriggerPort  VariantControl=(inherit)
  Gain : Gain  Gain=0.00001
  Memory : Memory  InheritSampleTime=on
  Subtract : Sum  Inputs=+-
  Out1 : Outport
  tau_n : Outport  Port=2
  wires:
  In1/1 -> Gain/1, Subtract/1, Memory/1
  Memory/1 -> Subtract/2
  Subtract/1 -> Out1/1
  Gain/1 -> tau_n/1

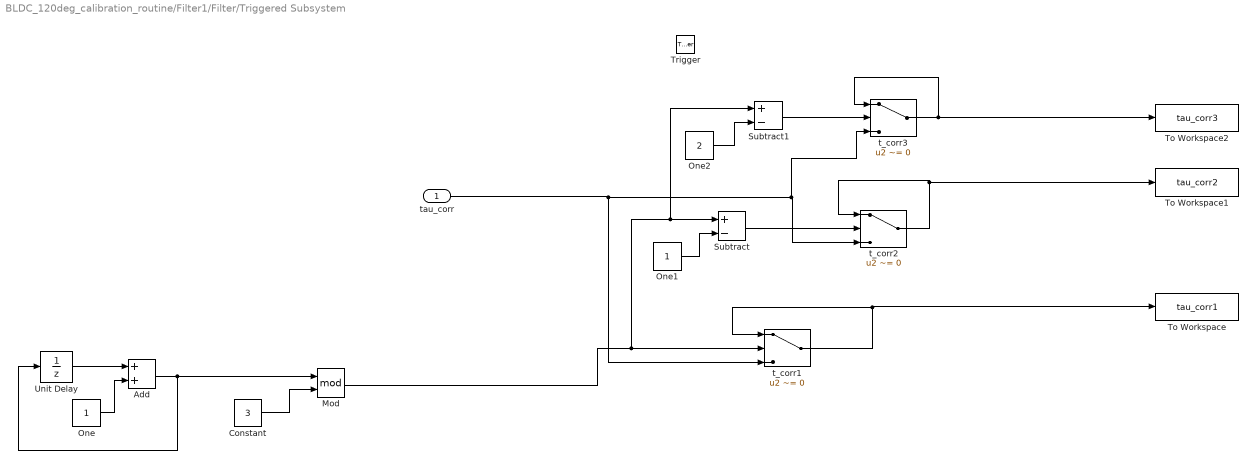
== system BLDC_120deg_calibration_routine/Filter1/Filter/Triggered Subsystem ==
  tau_corr : Inport
  Trigger : TriggerPort  VariantControl=(inherit)
  Add : Sum
  Constant : Constant  Value=3
  Mod : Math  Operator=mod
  One : Constant  OutDataTypeStr=Inherit: Inherit via back propagation
  One1 : Constant  OutDataTypeStr=Inherit: Inherit via back propagation
  One2 : Constant  Value=2  OutDataTypeStr=Inherit: Inherit via back propagation
  Subtract : Sum  Inputs=+-
  Subtract1 : Sum  Inputs=+-
  To Workspace : ToWorkspace  VariableName=tau_corr1  SampleTime=-1
  To Workspace1 : ToWorkspace  VariableName=tau_corr2  SampleTime=-1
  To Workspace2 : ToWorkspace  VariableName=tau_corr3  SampleTime=-1
  Unit Delay : UnitDelay  SampleTime=-1  HasFrameUpgradeWarning=on
  t_corr1 : Switch  Criteria=u2 ~= 0  SaturateOnIntegerOverflow=off  InputSameDT=off
  t_corr2 : Switch  Criteria=u2 ~= 0  SaturateOnIntegerOverflow=off  InputSameDT=off
  t_corr3 : Switch  Criteria=u2 ~= 0  SaturateOnIntegerOverflow=off  InputSameDT=off
  wires:
  Mod/1 -> Subtract1/1, Subtract/1, t_corr1/2
  Unit Delay/1 -> Add/1
  One/1 -> Add/2
  Add/1 -> Mod/1, Unit Delay/1
  Constant/1 -> Mod/2
  One1/1 -> Subtract/2
  Subtract/1 -> t_corr2/2
  One2/1 -> Subtract1/2
  Subtract1/1 -> t_corr3/2
  tau_corr/1 -> t_corr3/3, t_corr2/3, t_corr1/3
  t_corr1/1 -> To Workspace/1, t_corr1/1
  t_corr2/1 -> To Workspace1/1, t_corr2/1
  t_corr3/1 -> To Workspace2/1, t_corr3/1

== system BLDC_120deg_calibration_routine/Filter1/Filter/Triggered Subsystem1 ==
  Trigger : TriggerPort  VariantControl=(inherit)
  Subsystem : Subsystem  Priority=1
  Subsystem1 : Subsystem  Priority=2
  Subsystem2 : Subsystem  Priority=3
  Out3 : Outport
  Out2 : Outport  Port=2
  y : Outport  Port=3
  wires:
  Subsystem2/1(Out3) -> Out3/1
  Subsystem2/2(Out2) -> Out2/1
  Subsystem2/3(y) -> y/1

== system BLDC_120deg_calibration_routine/Filter1/Filter/Triggered Subsystem3 ==
  Trigger : TriggerPort  VariantControl=(inherit)
  Data Store Read : DataStoreRead  DataStoreName=hall_state  IndexOptions=Index vector (dialog)  Indices=1  OutputSizes=1
  Data Store Write : DataStoreWrite  DataStoreName=currHall  IndexOptions=Index vector (dialog)  Indices=1  OutputSizes=1
  wires:
  Data Store Read/1 -> Data Store Write/1

== system BLDC_120deg_calibration_routine/Filter1/Filter/Triggered Subsystem4 ==
  In1 : Inport
  tau-1 : Inport  Port=2
  tau-2 : Inport  Port=3
  tau-3 : Inport  Port=4
  tau-4 : Inport  Port=5
  tau-5 : Inport  Port=6
  Input3 : Inport  Port=7
  Trigger : TriggerPort  VariantControl=(inherit)
  Subsystem : Subsystem
  tau_corr : Outport
  Output : Outport  Port=2
  Output1 : Outport  Port=3
  wires:
  In1/1 -> Subsystem/1(In1)
  Subsystem/1(tau_corr) -> tau_corr/1
  tau-2/1 -> Subsystem/3(tau2)
  tau-3/1 -> Subsystem/4(tau3)
  tau-4/1 -> Subsystem/5(tau4)
  Input3/1 -> Subsystem/7(time)
  Subsystem/2(Output) -> Output/1
  Subsystem/3(Output1) -> Output1/1
  tau-1/1 -> Subsystem/2(tau-1)
  tau-5/1 -> Subsystem/6(tau-5)
